simulink library "fmr"  (Simulink 8.1)
settings: Solver=ode1  StartTime=0.0  StopTime=Inf  FixedStep=0.001  RelTol=1e-3
PostLoadFcn:
  | , if any(exist('dsrtsu_mdlpostloadfcn', 'file') == [2, 3, 6]), try dsrtsu_mdlpostloadfcn('Execute', bdroot); catch fprintf('Error in PostLoadFcn (dsrtsu_mdlpostloadfcn) for model "%s":\n %s\n', bdroot, lasterr); end, end,
undefined symbols (not defined in the file or in its folder): AACC_LowSpeedDistError_m, MACC_TargetSpeedMargin_mps
settings Model: DSRTSU_INTERNAL_RTI_VER=450  DSRTSU_INTERNAL_RTI_TYPE=rti1401  RTICANMMDATA=struct('GeneralSetupData',struct('modelroot','D:\ELN150201_TAIWAN\trunk\AdasDragon\software\sw_development\arch\app\acc','generalsettings',struct('filesettings',struct('destfolder',struct('Name','RTICANMM_FILES','Check',1),'buildfolder',struct('Name','.','Check',1),'AbsDestfolder',struct('Name','D:\ELN150201_TAIWAN\trunk\AdasDragon\software\sw_development\arch\app\acc\RTICANMM_FILES'),'AbsBuildfolder',struct('Name','D:\ELN150201_TAIWAN\trunk\AdasDragon\software\sw_development\arch\app\acc'))),'options',struct('addpaths',1,'rmpaths',1,'addtrcexclusion',logical(1),'cannavigator',struct('checkmonitoring',0),'show_usrtrc',0,'use_usrtrc',0),'advanced',struct('options',[1 1 1 1 1 1 1 1 1 1 1 1 1 1 1 1 1 1 1 1 1 1 1 1 1 1 1 1 1 1 1 1 1 1 1 1 1 1 1 1 1 1 1 1 1 1 1 1 1 1 1 1 1 1 1 1 1 1 1 1 1 1 1 1 1 1 1 1 1 1 1 1 1 1 1 1 1 1 1 1 1 1 1 1 1 1 1 1 1 1 1 1 1 1 1 1 1 1 1 1]),'MPSetup',{{}},'modelname','fmr','block','fmr'))  DSRTSU_INTERNAL_RTIFPGA=40  Creator=AT015411  LastModifiedBy=AT015555

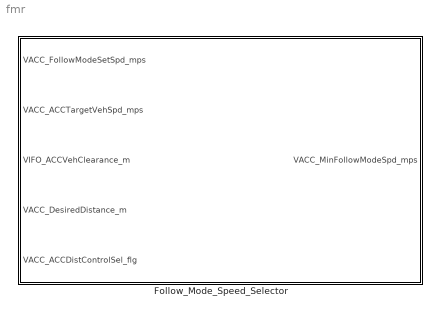
== system fmr ==
  Follow_Mode_Speed_Selector : Subsystem

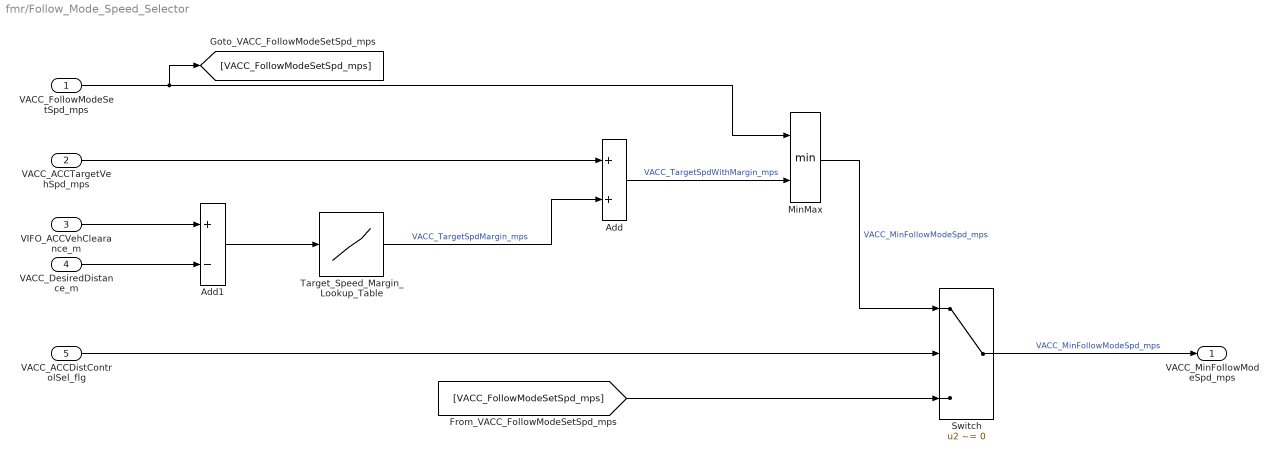
== system fmr/Follow_Mode_Speed_Selector ==
  VACC_FollowModeSetSpd_mps : Inport
  VACC_ACCTargetVehSpd_mps : Inport  Port=2
  VIFO_ACCVehClearance_m : Inport  Port=3
  VACC_DesiredDistance_m : Inport  Port=4
  VACC_ACCDistControlSel_flg : Inport  Port=5
  Add : Sum
  Add1 : Sum  Inputs=+-
  MinMax : MinMax  Inputs=2
  Switch : Switch  Criteria=u2 ~= 0
  Target_Speed_Margin_Lookup_Table : Lookup_n-D  NumberOfTableDimensions=1  BreakpointsForDimension1=AACC_LowSpeedDistError_m  Table=MACC_TargetSpeedMargin_mps  ExtrapMethod=Clip  UseLastTableValue=on  RndMeth=Simplest  InputSameDT=on
  VACC_MinFollowModeSpd_mps : Outport
  wires:
  [VACC_FollowModeSetSpd_mps] -> Switch/3
  MinMax/1 -> Switch/1  "VACC_MinFollowModeSpd_mps"
  VACC_ACCDistControlSel_flg/1 -> Switch/2
  Switch/1 -> VACC_MinFollowModeSpd_mps/1  "VACC_MinFollowModeSpd_mps"
  Add1/1 -> Target_Speed_Margin_Lookup_Table/1
  VACC_DesiredDistance_m/1 -> Add1/2
  VIFO_ACCVehClearance_m/1 -> Add1/1
  Target_Speed_Margin_Lookup_Table/1 -> Add/2  "VACC_TargetSpdMargin_mps"
  Add/1 -> MinMax/2  "VACC_TargetSpdWithMargin_mps"
  VACC_FollowModeSetSpd_mps/1 -> MinMax/1, [VACC_FollowModeSetSpd_mps]
  VACC_ACCTargetVehSpd_mps/1 -> Add/1
